simulink model "Modelo"  (R2021b)
settings: Solver=VariableStepAuto  StartTime=0.0  StopTime=10.0  RelTol=1e-3
undefined symbols (not defined in the file): bn, fn, ms
settings Model: Creator=alex_  LastModifiedBy=alex_

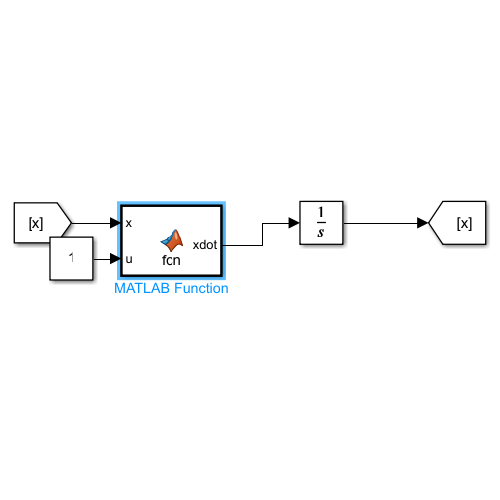
[thumbnail: Simulink's stored preview of the top-level diagram]
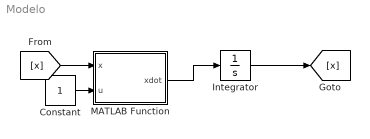
== system Modelo ==
  Constant : Constant
  Integrator : Integrator  InitialCondition=zeros(8,1)
  MATLAB Function : MATLAB Function  TreatAsAtomicUnit=on
  wires:
  MATLAB Function/1(xdot) -> Integrator/1
  Integrator/1 -> [x]
  [x] -> MATLAB Function/1(x)
  Constant/1 -> MATLAB Function/2(u)

== matlab function Modelo/MATLAB Function ==
  data: x input; u input; xdot output; fn parameter; bn parameter; ms parameter
function xdot  = fcn(x,u,fn, bn, ms)

I=eye(4);
Omega=diag(fn);
Zeta=diag(2*bn.*fn);


A=[zeros(4) I;
    -Omega -Zeta];

B=[zeros(4,1);
    ms'];

% C=[ms zeros(1,4)];
xdot=A*x+B*u;

% y=C*x;
